simulink subsystem "Push_button_to_Rolling_Buffer"  (R2023a)
settings: Solver=VariableStepAuto  StartTime=0.0  StopTime=10.0  RelTol=1e-3
libraries: dspsigops x1
settings Model: Creator=gcs_comp1  LastModifiedBy=gcs_comp1

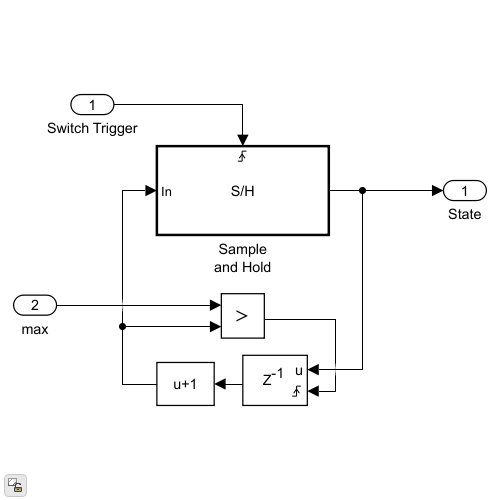
[thumbnail: Simulink's stored preview of the top-level diagram]
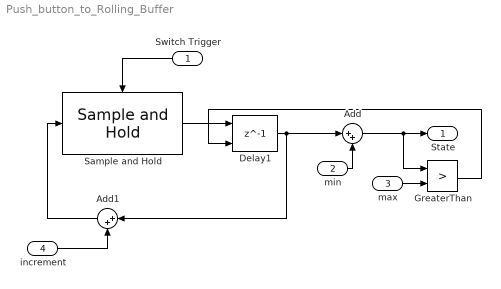
== system Push_button_to_Rolling_Buffer ==
  Switch Trigger : Inport
  min : Inport  Port=2
  max : Inport  Port=3
  increment : Inport  Port=4
  Add : Sum  Inputs=|++
  Add1 : Sum  Inputs=|++
  Delay1 : Delay  DelayLength=1  InitialCondition=0  ExternalReset=Rising
      settings: InputPortMap=u0,r5
  GreaterThan : RelationalOperator  Operator=>  OutDataTypeStr=boolean  RndMeth=Simplest  InputSameDT=off
  Sample and Hold : dspsigops/Sample and Hold  trig=Rising edge  initCond=0  latchinput=on
  State : Outport
  wires:
  Add1/1 -> Sample and Hold/1
  Switch Trigger/1 -> Sample and Hold/Trigger
  max/1 -> GreaterThan/2
  Add/1 -> State/1, GreaterThan/1
  min/1 -> Add/2
  Delay1/1 -> Add/1, Add1/1
  GreaterThan/1 -> Delay1/2
  Sample and Hold/1 -> Delay1/1
  increment/1 -> Add1/2
